simulink model "BLDCmotor_modeling"  (R2015b)
settings: Solver=VariableStepAuto  StartTime=0.0  StopTime=10  RelTol=1e-3
values from neighbouring files (symbols this model uses):
  B = 0.1    [BLDCmotor_modeling_param.m]    (also in DCmotor_modeling_ss.m = [1/L; 0; 0])
  J = 0.1    [BLDCmotor_modeling_param.m]    (also in DCmotor_modeling_ss.m = 0.02)
  L = 0.1    [BLDCmotor_modeling_param.m]    (also in DCmotor_modeling_ss.m = 0.5)
  P = 30    [BLDCmotor_modeling_param.m]
  R = 0.02    [BLDCmotor_modeling_param.m]    (also in DCmotor_modeling_ss.m = 2)
undefined symbols (not defined in the file or in its folder): ke, kt, trapezoid
settings Model: Creator=weberhsu  LastModifiedBy=root

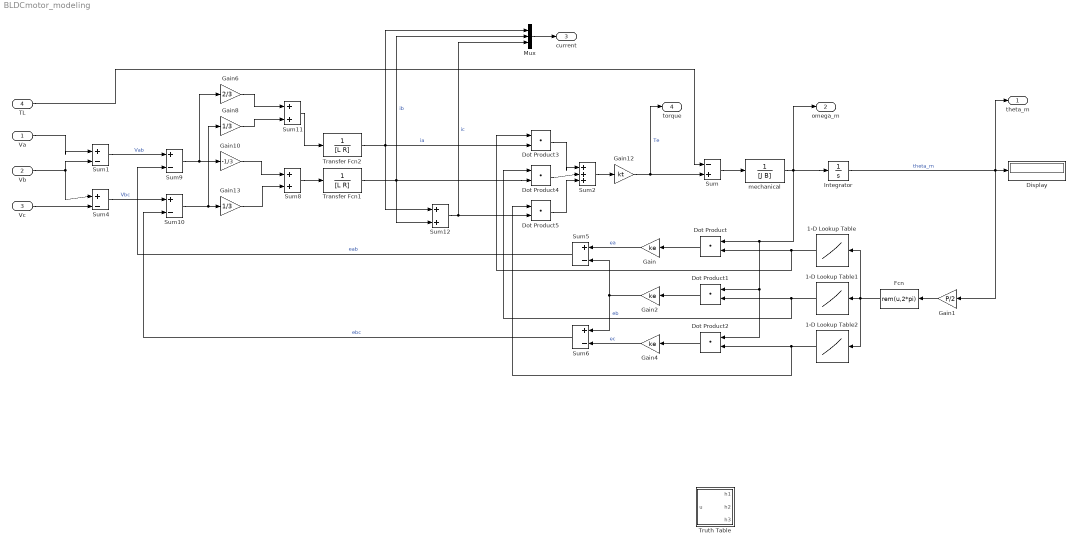
== system BLDCmotor_modeling ==
  Va : Inport
  Vb : Inport  Port=2
  Vc : Inport  Port=3
  TL : Inport  Port=4
  1-D Lookup Table : Lookup_n-D  NumberOfTableDimensions=1  BreakpointsForDimension1=0:0.1:2*pi  Table=trapezoid(0:0.1:2*pi,0)  InternalRulePriority=Speed  RndMeth=Simplest  InputSameDT=on
  1-D Lookup Table1 : Lookup_n-D  NumberOfTableDimensions=1  BreakpointsForDimension1=((0:0.1:2*pi))  Table=trapezoid(0:0.1:2*pi, 2/3*pi)  InternalRulePriority=Speed  RndMeth=Simplest  InputSameDT=on
  1-D Lookup Table2 : Lookup_n-D  NumberOfTableDimensions=1  BreakpointsForDimension1=(0:0.1:2*pi)  Table=trapezoid(0:0.1:2*pi, 4/3*pi)  InternalRulePriority=Speed  RndMeth=Simplest  InputSameDT=on
  Display : Display
  Dot Product{,1..5} (6 alike) : DotProduct  InputSameDT=on  OutDataTypeStr=Inherit: Inherit via internal rule
  Fcn : Fcn  Expr=rem(u,2*pi)
  Gain : Gain  Gain=ke
  Gain1 : Gain  Gain=P/2
  Gain10 : Gain  Gain=-1/3
  Gain12 : Gain  Gain=kt
  Gain13 : Gain  Gain=1/3
  Gain2 : Gain  Gain=ke
  Gain4 : Gain  Gain=ke
  Gain6 : Gain  Gain=2/3
  Gain8 : Gain  Gain=1/3
  Integrator : Integrator
  Mux : Mux  Inputs=3
  Sum : Sum  Inputs=-+
  Sum1 : Sum  Inputs=|+-
  Sum{5..6,9..10} (4 alike) : Sum  Inputs=+-
  Sum11 : Sum
  Sum12 : Sum
  Sum2 : Sum  Inputs=|+++
  Sum4 : Sum  Inputs=|+-
  Sum8 : Sum
  Transfer Fcn1 : TransferFcn  Denominator=[L R]
  Transfer Fcn2 : TransferFcn  Denominator=[L R]
  Truth Table : Truth Table  TreatAsAtomicUnit=on
  mechanical : TransferFcn  Denominator=[J B]
  theta_m : Outport
  omega_m : Outport  Port=2
  current : Outport  Port=3
  torque : Outport  Port=4
  wires:
  mechanical/1 -> omega_m/1, Integrator/1, Dot Product2/1, Dot Product1/1, Dot Product/1
  Integrator/1 -> theta_m/1, Display/1, Gain1/1  "theta_m"
  Sum/1 -> mechanical/1
  Gain12/1 -> torque/1, Sum/2  "Te"
  Sum2/1 -> Gain12/1
  Dot Product3/1 -> Sum2/1
  Dot Product4/1 -> Sum2/2
  Dot Product5/1 -> Sum2/3
  Va/1 -> Sum1/1
  Vb/1 -> Sum4/1, Sum1/2
  Vc/1 -> Sum4/2
  Sum1/1 -> Sum9/1  "Vab"
  Sum4/1 -> Sum10/1  "Vbc"
  Gain/1 -> Sum5/1  "ea"
  Gain2/1 -> Sum6/1, Sum5/2  "eb"
  Gain4/1 -> Sum6/2  "ec"
  Sum5/1 -> Sum9/2  "eab"
  Sum6/1 -> Sum10/2  "ebc"
  Gain10/1 -> Sum8/1
  Sum8/1 -> Transfer Fcn1/1
  Transfer Fcn1/1 -> Dot Product4/2, Mux/2, Sum12/2  "ib"
  Sum9/1 -> Gain10/1, Gain6/1
  Sum10/1 -> Gain8/1, Gain13/1
  Transfer Fcn2/1 -> Mux/1, Dot Product3/2, Sum12/1  "ia"
  Gain6/1 -> Sum11/1
  Gain8/1 -> Sum11/2
  Sum11/1 -> Transfer Fcn2/1
  Sum12/1 -> Mux/3, Dot Product5/2  "ic"
  Gain13/1 -> Sum8/2
  1-D Lookup Table/1 -> Dot Product/2, Dot Product3/1
  Dot Product/1 -> Gain/1
  1-D Lookup Table1/1 -> Dot Product1/2, Dot Product4/1
  1-D Lookup Table2/1 -> Dot Product2/2, Dot Product5/1
  Dot Product1/1 -> Gain2/1
  Dot Product2/1 -> Gain4/1
  Gain1/1 -> Fcn/1
  Fcn/1 -> 1-D Lookup Table2/1, 1-D Lookup Table1/1, 1-D Lookup Table/1
  TL/1 -> Sum/1
  Mux/1 -> current/1

== matlab function BLDCmotor_modeling/Truth Table ==
  data: u input; h1 output; h2 output; h3 output
function [h1,h2, h3] = fcn(u)

aVarTruthTableCondition_1 = false;
aVarTruthTableCondition_2 = false;


% Example condition 1

aVarTruthTableCondition_1 = logical(u >= 0);

% Example condition 2

aVarTruthTableCondition_2 = logical(u ^ 2 <= 1);

if (aVarTruthTableCondition_1 && aVarTruthTableCondition_2)
    aFcnTruthTableAction_1();
elseif (~aVarTruthTableCondition_1 && ~aVarTruthTableCondition_2)
    aFcnTruthTableAction_1();
else % Default
    aFcnTruthTableAction_2();
end

function aFcnTruthTableAction_1()

% Example action 1 called from D1 & D2 column in condition table

y = u;

function aFcnTruthTableAction_2()

% Example action 2 called from D3 column in condition table

y = 1 / u;
